simulink model "Bicycle_PID2"  (R2024b)
settings: Solver=ode4  StartTime=0.0  StopTime=150  FixedStep=0.02  MaxStep=0.05  RelTol=1e-3
InitFcn:
  | clear persistent_anim_update
  | clear nearest_ref_point
values from neighbouring files (symbols this model uses):
  theta_init = theta_ref_arr(closest_idx)    [PIDScript2.m]
  x_init = sp(1)    [PIDScript2.m]
  y_init = sp(2)    [PIDScript2.m]
libraries: slpidlib x2
settings Model: PacingRate=1.300000  Creator=kasimesen  LastModifiedBy=kasimesen
settings DataIOCC: ReturnWorkspaceOutputs=off

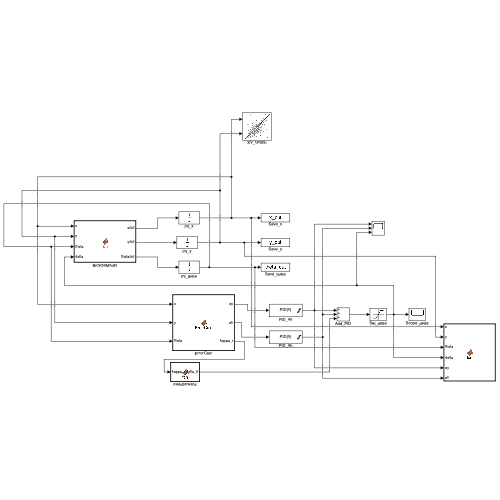
[thumbnail: Simulink's stored preview of the top-level diagram]
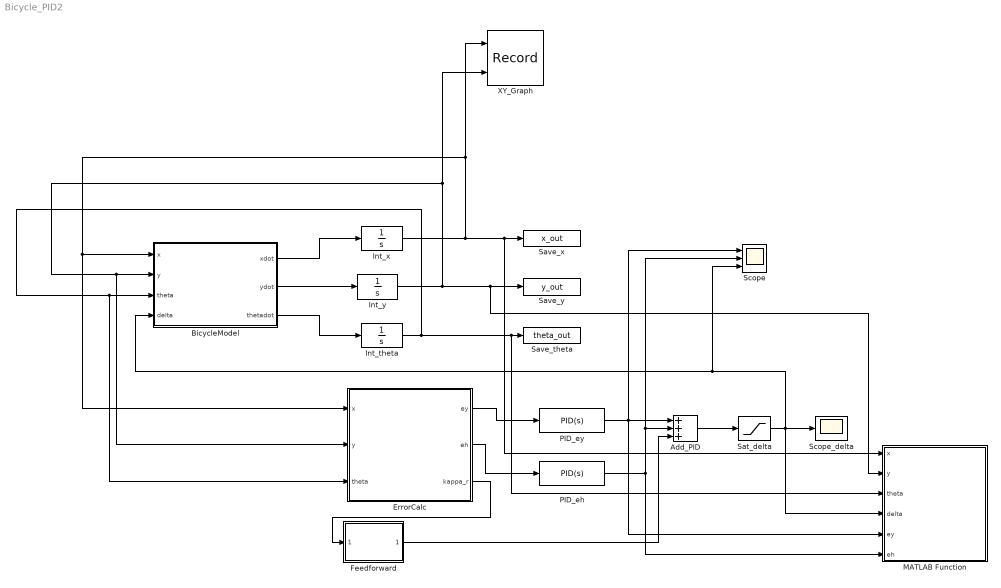
== system Bicycle_PID2 ==
  Add_PID : Sum  Inputs=+++
  BicycleModel : MATLAB Function  TreatAsAtomicUnit=on
  ErrorCalc : MATLAB Function  TreatAsAtomicUnit=on
  Feedforward : MATLAB Function  TreatAsAtomicUnit=on
  Int_theta : Integrator  InitialCondition=theta_init
  Int_x : Integrator  InitialCondition=x_init
  Int_y : Integrator  InitialCondition=y_init
  MATLAB Function : MATLAB Function  TreatAsAtomicUnit=on
  PID_eh : slpidlib/PID Controller  Controller=PID  Form=Parallel  TimeDomain=Continuous-time  UseExternalTs=off  SampleTime=-1  IntegratorMethod=Forward Euler  FilterMethod=Forward Euler  ControllerParametersSource=internal  P=-7.0  I=-0.2  UseKiTs=off  D=0.0  UseExternalDerivativeSource=off  N=100  UseFilter=on  TunerSelectOption=Transfer Function Based (PID Tuner App)  InitialConditionSource=internal  InitialConditionForIntegrator=0  InitialConditionForFilter=0  DifferentiatorICPrevScaledInput=0  ExternalReset=none  TrackingMode=off  Kt=1  LimitOutput=on  SatLimitsSource=internal  UpperSaturationLimit=0.25  LowerSaturationLimit=-0.25  LinearizeAsGain=on  AntiWindupMode=clamping  Kb=1  LimitIntegrator=off  UpperIntegratorSaturationLimit=inf  LowerIntegratorSaturationLimit=-inf  POutMin=[]  POutMax=[]  IOutMin=[]  IOutMax=[]  DOutMin=[]  DOutMax=[]  NOutMin=[]  NOutMax=[]  SumOutMin=[]  SumOutMax=[]  SaturationOutMin=[]  SaturationOutMax=[]  PParamMin=[]  PParamMax=[]  IParamMin=[]  IParamMax=[]  DParamMin=[]  DParamMax=[]  NParamMin=[]  NParamMax=[]  KbParamMin=[]  KbParamMax=[]  KtParamMin=[]  KtParamMax=[]  KbOutMin=[]  KbOutMax=[]  KtOutMin=[]  KtOutMax=[]  IntegratorOutMin=[]  IntegratorOutMax=[]  FilterOutMin=[]  FilterOutMax=[]  SumI1OutMin=[]  SumI1OutMax=[]  SumI2OutMin=[]  SumI2OutMax=[]  SumI3OutMin=[]  SumI3OutMax=[]  SumI4OutMin=[]  SumI4OutMax=[]  SumDOutMin=[]  SumDOutMax=[]  DifferentiatorOutMin=[]  DifferentiatorOutMax=[]  FilterDiffOutCoefMin=[]  FilterDiffOutCoefMax=[]  ReciprocalOutMin=[]  ReciprocalOutMax=[]  SumDenOutMin=[]  SumDenOutMax=[]  SumNumOutMin=[]  SumNumOutMax=[]  DivideOutMin=[]  DivideOutMax=[]  UdiffTsProdOutMin=[]  UdiffTsProdOutMax=[]  NTsProdOutMin=[]  NTsProdOutMax=[]  UintegralTsProdOutMin=[]  UintegralTsProdOutMax=[]  UngainTsProdOutMin=[]  UngainTsProdOutMax=[]  ClampingZeroOutDataTypeStr=Inherit: Inherit via back propagation  ClampingZeroOutMin=[]  ClampingZeroOutMax=[]  FilterDenConstantOutDataTypeStr=Inherit: Inherit via back propagation  FilterDenConstantOutMin=[]  FilterDenConstantOutMax=[]  PCopyOutDataTypeStr=Inherit: Inherit via back propagation  PCopyOutMin=[]  PCopyOutMax=[]  NCopyOutDataTypeStr=Inherit: Inherit via back propagation  NCopyOutMin=[]  NCopyOutMax=[]  IntegratorContinuousStateAttributes=''  IntegratorStateMustResolveToSignalObject=off  IntegratorRTWStateStorageClass=Auto  FilterContinuousStateAttributes=''  FilterStateMustResolveToSignalObject=off  FilterRTWStateStorageClass=Auto  ParallelPVariant=InternalParameters  IdealPVariant=Disabled  IVariant=InternalParameters  DVariant=InternalParameters  IntegratorVariant=Continuous  SatVariant=Enabled  AWVariant=ContClampingParallel  PCopyVariant=Disabled  TRVariant=Disabled  FdbkBlocksVariant=Forward  IdealPFdbkVariant=Disabled  SatFdbkVariant=Disabled  DerivativeFilterVariant=ContFilter  NVariant=InternalParameters  NCopyVariant=Disabled  FilterICVariant=InternalICsFilter  IntegratorICVariant=InternalICs  ExternalResetVariant=Disabled  TRSumVariant=Passthrough  SumFdbkVariant=Disabled  SumVariant=Sum_PID  TsampFilterVariant=InternalTs  TsampNgainVariant=Passthrough  TsampIntegralVariant=Disabled_SignalSpec  ExternalSaturationOutDataTypeStr=Inherit: Same as second input  DerivativeSourceVariant=ErrorSignal  PreIntVariant=InternalPreInt
  PID_ey : slpidlib/PID Controller  Controller=PID  Form=Parallel  TimeDomain=Continuous-time  UseExternalTs=off  SampleTime=-1  IntegratorMethod=Forward Euler  FilterMethod=Forward Euler  ControllerParametersSource=internal  P=-14.0  I=-0.4  UseKiTs=off  D=0.0  UseExternalDerivativeSource=off  N=100  UseFilter=on  TunerSelectOption=Transfer Function Based (PID Tuner App)  InitialConditionSource=internal  InitialConditionForIntegrator=0  InitialConditionForFilter=0  DifferentiatorICPrevScaledInput=0  ExternalReset=none  TrackingMode=off  Kt=1  LimitOutput=on  SatLimitsSource=internal  UpperSaturationLimit=0.35  LowerSaturationLimit=-0.35  LinearizeAsGain=on  AntiWindupMode=clamping  Kb=1  LimitIntegrator=off  UpperIntegratorSaturationLimit=inf  LowerIntegratorSaturationLimit=-inf  POutMin=[]  POutMax=[]  IOutMin=[]  IOutMax=[]  DOutMin=[]  DOutMax=[]  NOutMin=[]  NOutMax=[]  SumOutMin=[]  SumOutMax=[]  SaturationOutMin=[]  SaturationOutMax=[]  PParamMin=[]  PParamMax=[]  IParamMin=[]  IParamMax=[]  DParamMin=[]  DParamMax=[]  NParamMin=[]  NParamMax=[]  KbParamMin=[]  KbParamMax=[]  KtParamMin=[]  KtParamMax=[]  KbOutMin=[]  KbOutMax=[]  KtOutMin=[]  KtOutMax=[]  IntegratorOutMin=[]  IntegratorOutMax=[]  FilterOutMin=[]  FilterOutMax=[]  SumI1OutMin=[]  SumI1OutMax=[]  SumI2OutMin=[]  SumI2OutMax=[]  SumI3OutMin=[]  SumI3OutMax=[]  SumI4OutMin=[]  SumI4OutMax=[]  SumDOutMin=[]  SumDOutMax=[]  DifferentiatorOutMin=[]  DifferentiatorOutMax=[]  FilterDiffOutCoefMin=[]  FilterDiffOutCoefMax=[]  ReciprocalOutMin=[]  ReciprocalOutMax=[]  SumDenOutMin=[]  SumDenOutMax=[]  SumNumOutMin=[]  SumNumOutMax=[]  DivideOutMin=[]  DivideOutMax=[]  UdiffTsProdOutMin=[]  UdiffTsProdOutMax=[]  NTsProdOutMin=[]  NTsProdOutMax=[]  UintegralTsProdOutMin=[]  UintegralTsProdOutMax=[]  UngainTsProdOutMin=[]  UngainTsProdOutMax=[]  ClampingZeroOutDataTypeStr=Inherit: Inherit via back propagation  ClampingZeroOutMin=[]  ClampingZeroOutMax=[]  FilterDenConstantOutDataTypeStr=Inherit: Inherit via back propagation  FilterDenConstantOutMin=[]  FilterDenConstantOutMax=[]  PCopyOutDataTypeStr=Inherit: Inherit via back propagation  PCopyOutMin=[]  PCopyOutMax=[]  NCopyOutDataTypeStr=Inherit: Inherit via back propagation  NCopyOutMin=[]  NCopyOutMax=[]  IntegratorContinuousStateAttributes=''  IntegratorStateMustResolveToSignalObject=off  IntegratorRTWStateStorageClass=Auto  FilterContinuousStateAttributes=''  FilterStateMustResolveToSignalObject=off  FilterRTWStateStorageClass=Auto  ParallelPVariant=InternalParameters  IdealPVariant=Disabled  IVariant=InternalParameters  DVariant=InternalParameters  IntegratorVariant=Continuous  SatVariant=Enabled  AWVariant=ContClampingParallel  PCopyVariant=Disabled  TRVariant=Disabled  FdbkBlocksVariant=Forward  IdealPFdbkVariant=Disabled  SatFdbkVariant=Disabled  DerivativeFilterVariant=ContFilter  NVariant=InternalParameters  NCopyVariant=Disabled  FilterICVariant=InternalICsFilter  IntegratorICVariant=InternalICs  ExternalResetVariant=Disabled  TRSumVariant=Passthrough  SumFdbkVariant=Disabled  SumVariant=Sum_PID  TsampFilterVariant=InternalTs  TsampNgainVariant=Passthrough  TsampIntegralVariant=Disabled_SignalSpec  ExternalSaturationOutDataTypeStr=Inherit: Same as second input  DerivativeSourceVariant=ErrorSignal  PreIntVariant=InternalPreInt
  Sat_delta : Saturate  UpperLimit=0.5236  LowerLimit=-0.5236
  Save_theta : ToWorkspace  VariableName=theta_out  SaveFormat=Timeseries  SampleTime=-1
  Save_x : ToWorkspace  VariableName=x_out  SaveFormat=Timeseries  SampleTime=-1
  Save_y : ToWorkspace  VariableName=y_out  SaveFormat=Timeseries  SampleTime=-1
  Scope : Scope  NumInputPorts=3
  Scope_delta : Scope
  XY_Graph : Record  FileSettingsInternal="{\"entries\":[{\"content\":{\"excelSettings\":{\"content\":{},\"type\":\"Streamout.ExcelSettings\"}},\"type\":\"Streamout.FileSettingStorage\",\"uuid\":\"\"}],\"packageUris\":[\"http:\\/\\/schema.mathworks.com\\/mf0\\/streamout_blocks\\/R2020a\"],\"version\":\"1.0\"}"  Layout=[1 1]  SignalsInternal="{\"entries\":[{\"content\":{\"signals\":[{\"content\":{\"blockPath\":[],\"dimensions\":[1],\"domain\":\"\",\"lineColor\":\"#a2142f\",\"plots\":[ 1 ],\"port\":1,\"sid\":[\"\"],\"signalID\":1,\"signalName\":\"Int_x\"},\"type\":\"RecordBlkView.Signal\",\"uuid\":\"\"},{\"content\":{\"blockPath\":[],\"dimensions\":[1],\"domain\":\"\",\"lineColor\":\"#139fff\",\"plots\":[ 1 ],\"port\":2,\"sid\":[\"\"],\"signalID\":2,\"signalName\":\"Int_y\"},\"type\":\"RecordBlkView.Signal\",\"uuid\":\"\"}]},\"type\":\"RecordBlkView.InputSignals\",\"uuid\":\"\"}],\"packageUris\":[\"http:\\/\\/schema.mathworks.com\\/mf0\\/streamout_blocks\\/R2020a\"],\"version\":\"1.0\"}"  VisualizationBindings="{\"xyplotplugin\":{\"info\":[{\"series\":[{\"bindingParametersList\":[{\"parameter\":\"X-Axis\",\"signalID\":1,\"signalName\":\"Int_x\"},{\"parameter\":\"Y-Axis\",\"signalID\":2,\"signalName\":\"Int_y\"}],\"seriesID\":0}],\"subplotID\":1}]}}"  CompatibilityTag=XY
  wires:
  ErrorCalc/1(ey) -> PID_ey/1
  ErrorCalc/2(eh) -> PID_eh/1
  PID_eh/1 -> MATLAB Function/6(eh), Scope/2, Add_PID/2
  PID_ey/1 -> MATLAB Function/5(ey), Scope/1, Add_PID/1
  Add_PID/1 -> Sat_delta/1
  Sat_delta/1 -> MATLAB Function/4(delta), Scope/3, BicycleModel/4(delta), Scope_delta/1
  BicycleModel/1(xdot) -> Int_x/1
  BicycleModel/2(ydot) -> Int_y/1
  BicycleModel/3(thetadot) -> Int_theta/1
  Int_x/1 -> MATLAB Function/1(x), Save_x/1, ErrorCalc/1(x), BicycleModel/1(x), XY_Graph/1
  Int_y/1 -> ErrorCalc/2(y), BicycleModel/2(y), XY_Graph/2, MATLAB Function/2(y), Save_y/1
  Int_theta/1 -> MATLAB Function/3(theta), Save_theta/1, ErrorCalc/3(theta), BicycleModel/3(theta)
  Feedforward/1(delta_ff) -> Add_PID/3
  ErrorCalc/3(kappa_r) -> Feedforward/1(kappa_r)

== matlab function Bicycle_PID2/BicycleModel ==
  data: x input; xdot output; y input; theta input; delta input; ydot output; thetadot output
function [xdot, ydot, thetadot] = fcn(x, y, theta, delta)
% BICYCLE KINEMATIC MODEL (CONTINUOUS)
%
% Girişler: x, y, theta (araç durumu), delta (direksiyon)
% Çıkışlar: xdot, ydot, thetadot

L     = 2.7;    % Dingil mesafesi (m)
lr    = 1.35;    % Arka aks - kütle merkezine uzaklık (m)
v_ref = 8.0;    % Referans hız (m/s)

% Slip angle
beta = atan((lr/L) * tan(delta));

% Kinematik denklemler
xdot     = v_ref * cos(theta + beta);
ydot     = v_ref * sin(theta + beta);
thetadot = (v_ref/L) * cos(beta) * tan(delta);
end

== matlab function Bicycle_PID2/ErrorCalc ==
  data: x input; ey output; y input; theta input; eh output; kappa_r output
function [ey, eh, kappa_r] = ErrorCalc(x, y, theta)
% PID HATA HESABI

coder.extrinsic('nearest_ref_point');

xr  = 0;
yr  = 0;
thr = 0;
kappa_r = 0;

[xr, yr, thr, kappa_r] = nearest_ref_point(x, y);

approach_dist = 20.0;

dist = sqrt((x - xr)^2 + (y - yr)^2);

if dist >= approach_dist
    % UZAK: hedefe doğru git
    desired = atan2(yr - y, xr - x);
    ey = 0;
    eh = mod(theta - desired + pi, 2*pi) - pi;
else
    % YAKIN: saf PID
    ex = x - xr;
    ey = -sin(thr)*ex + cos(thr)*(y - yr);
    eh = mod(theta - thr + pi, 2*pi) - pi;
end
end

== matlab function Bicycle_PID2/MATLAB Function ==
  data: x input; y input; theta input; delta input; ey input; eh input
function fcn(x, y, theta, delta, ey, eh)
% ANİMASYON
% Referans yolu workspace'ten okur.

coder.extrinsic('persistent_anim_update');
persistent_anim_update(x, y, theta, delta, ey, eh);
end

== matlab function Bicycle_PID2/Feedforward ==
  data: kappa_r input; delta_ff output
function delta_ff = fcn(kappa_r)

L = 2.7;

delta_ff = atan(L * kappa_r);

end
